simulink model "Simulink_simulation"  (R2023a)
settings: Solver=VariableStepAuto  StartTime=0.0  StopTime=20  MaxStep=0.01  RelTol=1e-3
InitFcn:
  | %init
values from neighbouring files (symbols this model uses):
  K = 1    [init.m]
  k1 = 1    [init.m]
  k2 = 1    [init.m]
  k_omega = 1    [init.m]
  k_v = 1    [init.m]
  lambda2 = 0.5    [init.m]
  q0 = [sqrt(qinit(1)^2+qinit(2)); atan(qinit(2)/qinit(1)) - pi; atan(qinit(2)/qinit(1)) - pi - qinit(3)]    [init.m]
  q_final = [0; 0; 0]    [init.m]
  t_omega = t_v    (= 0.8)    [init.m]
  t_v = 0.8    [init.m]
settings Model: Creator=rvitt  LastModifiedBy=rvitt
settings OptimizationCC: ReuseModelBlockBuffer=off

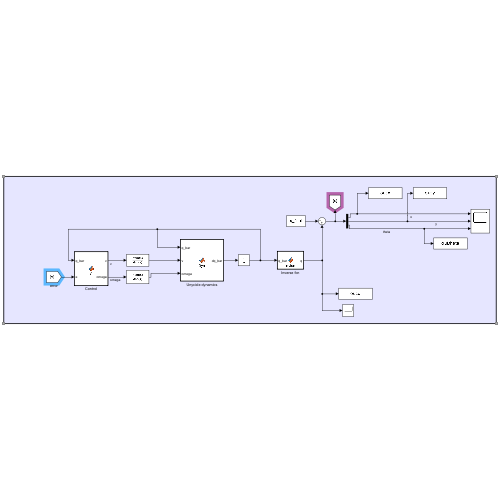
[thumbnail: Simulink's stored preview of the top-level diagram]
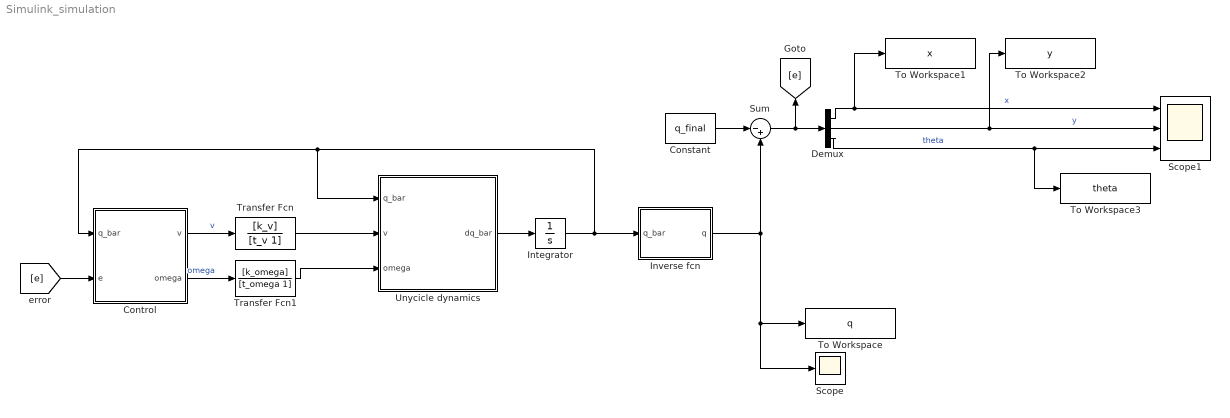
== system Simulink_simulation ==
  Constant : Constant  Value=q_final
  Control : MATLAB Function  TreatAsAtomicUnit=on
  Demux : Demux  Outputs=3
  Integrator : Integrator  InitialCondition=q0
  Inverse fcn : MATLAB Function  TreatAsAtomicUnit=on
  Scope : Scope
  Scope1 : Scope  NumInputPorts=3
  Sum : Sum  Inputs=|-+
  To Workspace : ToWorkspace  VariableName=q  SaveFormat=Timeseries  SampleTime=-1
  To Workspace1 : ToWorkspace  VariableName=x  SaveFormat=Timeseries  SampleTime=-1
  To Workspace2 : ToWorkspace  VariableName=y  SaveFormat=Timeseries  SampleTime=-1
  To Workspace3 : ToWorkspace  VariableName=theta  SaveFormat=Timeseries  SampleTime=-1
  Transfer Fcn : TransferFcn  Numerator=[k_v]  Denominator=[t_v 1]
  Transfer Fcn1 : TransferFcn  Numerator=[k_omega]  Denominator=[t_omega 1]
  Unycicle dynamics : MATLAB Function  TreatAsAtomicUnit=on
  wires:
  Unycicle dynamics/1(dq_bar) -> Integrator/1
  Integrator/1 -> Unycicle dynamics/1(q_bar), Control/1(q_bar), Inverse fcn/1(q_bar)
  Control/2(omega) -> Transfer Fcn1/1  "omega"
  Control/1(v) -> Transfer Fcn/1  "v"
  Inverse fcn/1(q) -> Scope/1, To Workspace/1, Sum/2
  Transfer Fcn/1 -> Unycicle dynamics/2(v)
  Constant/1 -> Sum/1
  Sum/1 -> [e], Demux/1
  Demux/2 -> To Workspace2/1, Scope1/2  "y"
  Demux/3 -> To Workspace3/1, Scope1/3  "theta"
  Demux/1 -> To Workspace1/1, Scope1/1  "x"
  Transfer Fcn1/1 -> Unycicle dynamics/3(omega)
  [e] -> Control/2(e)

== matlab function Simulink_simulation/Control ==
  data: q_bar input; e input; v output; omega output; k1 parameter; k2 parameter; lambda2 parameter; K parameter
function [v, omega] = C(q_bar, e, k1, k2, lambda2, K)

% State variable
rho = q_bar(1);
phi = q_bar(2);
alpha = q_bar(3);

% v = k1*cos(alpha)*rho;
%     omega = k2*sin(alpha)/alpha*cos(alpha)*(alpha + lambda2*phi) + k2*alpha;

% 2 step control
if e(1) > 0.01 || e(2) > 0.01
    v = k1*cos(alpha)*rho;
    omega = k2*sin(alpha)/alpha*cos(alpha)*(alpha + lambda2*phi) + k2*alpha;
    
else
    v = 0;
    omega = -K*e(3);
end

== matlab function Simulink_simulation/Unycicle dynamics ==
  data: q_bar input; v input; dq_bar output; omega input
function dq_bar = Dyn(q_bar, v, omega)

% Rename variables
rho = q_bar(1);
phi = q_bar(2);
alpha = q_bar(3);

% Input in bar state variable
w = v/rho;

% System dynamics in alternative variables
dq_bar = [-rho*cos(alpha); sin(alpha); sin(alpha)]*w + [0; 0; -1]*omega;

== matlab function Simulink_simulation/Inverse fcn ==
  data: q_bar input; q output; q_final parameter
function q = invfcn(q_bar, q_final)

% Rename variables
rho = q_bar(1);
phi = q_bar(2);
alpha = q_bar(3);

% Inv funcition
q = [-rho*cos(phi); -rho*sin(phi); phi-alpha] + q_final;
